simulink model "smc"  (R2022b)
settings: Solver=VariableStepAuto  StartTime=0.0  StopTime=10
undefined symbols (not defined in the file or in its folder): a, beta, d1, d2, delta, DZ, I, km, miu, wb, wcp, wm
settings Model: Creator=andre  LastModifiedBy=felip
settings SolverCC: ZeroCrossAlgorithm=Adaptive  AlgebraicLoopSolver=TrustRegion
settings DebuggingCC: IgnoredZcDiagnostic=none  UnconnectedInputMsg=warning  UnconnectedOutputMsg=warning  UnconnectedLineMsg=warning  SFMachineParentedDataDiag=warning
settings ModelReferenceCC: EnableRefExpFcnMdlSchedulingChecks=on
settings RTWCC: DLArmComputeVersion=19.05

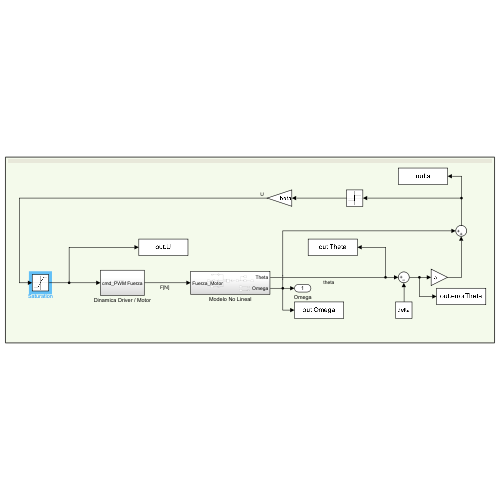
[thumbnail: Simulink's stored preview of the top-level diagram]
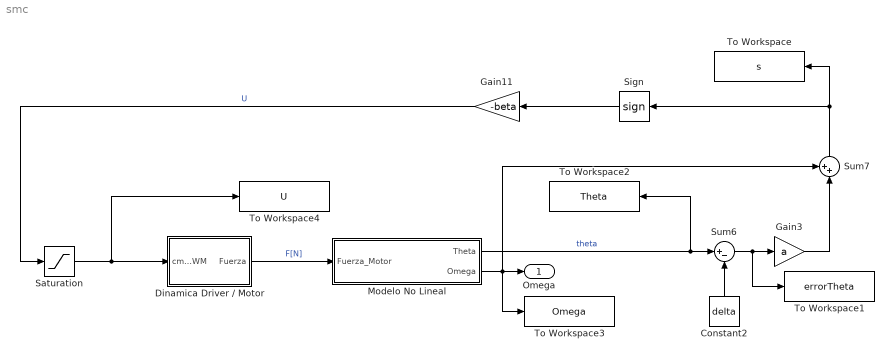
== system smc ==
  Constant2 : Constant  Value=delta
  Dinamica Driver / Motor : Subsystem
  Gain11 : Gain  Gain=-beta
  Gain3 : Gain  Gain=a
  Modelo No Lineal : Subsystem
  Saturation : Saturate  UpperLimit=95  LowerLimit=5  ZeroCross=off
  Sign : Signum  ZeroCross=off
  Sum6 : Sum  Inputs=|+-
  Sum7 : Sum  Inputs=++|
  To Workspace : ToWorkspace  VariableName=s  SaveFormat=Timeseries  SampleTime=-1
  To Workspace1 : ToWorkspace  VariableName=errorTheta  SaveFormat=Timeseries  SampleTime=-1
  To Workspace2 : ToWorkspace  VariableName=Theta  SaveFormat=Timeseries  SampleTime=-1
  To Workspace3 : ToWorkspace  VariableName=Omega  SaveFormat=Timeseries  SampleTime=-1
  To Workspace4 : ToWorkspace  VariableName=U  SaveFormat=Timeseries  SampleTime=-1
  Omega : Outport
  wires:
  Gain3/1 -> Sum7/2
  Modelo No Lineal/1(Theta) -> To Workspace2/1, Sum6/1  "theta"
  Sum7/1 -> To Workspace/1, Sign/1
  Gain11/1 -> Saturation/1  "U"
  Constant2/1 -> Sum6/2
  Dinamica Driver / Motor/1(Fuerza) -> Modelo No Lineal/1(Fuerza_Motor)  "F[N]"
  Modelo No Lineal/2(Omega) -> To Workspace3/1, Omega/1, Sum7/1
  Saturation/1 -> To Workspace4/1, Dinamica Driver / Motor/1(cmd_PWM)
  Sign/1 -> Gain11/1
  Sum6/1 -> To Workspace1/1, Gain3/1

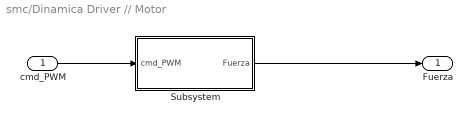
== system smc/Dinamica Driver // Motor ==
  cmd_PWM : Inport
  Subsystem : Subsystem
  Fuerza : Outport
  wires:
  Subsystem/1(Fuerza) -> Fuerza/1
  cmd_PWM/1 -> Subsystem/1(cmd_PWM)

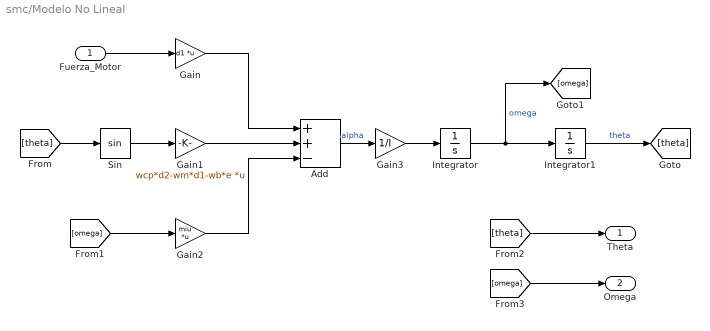
== system smc/Modelo No Lineal ==
  Fuerza_Motor : Inport
  Add : Sum  Inputs=++-
  Gain : Gain  Gain=d1  Multiplication=Matrix(K*u)
  Gain1 : Gain  Gain=wcp*d2-wm*d1-wb*e  Multiplication=Matrix(K*u)
  Gain2 : Gain  Gain=miu  Multiplication=Matrix(K*u)
  Gain3 : Gain  Gain=1/I
  Integrator : Integrator  ZeroCross=off
  Integrator1 : Integrator  ZeroCross=off
  Sin : Trigonometry  ApproximationMethod=CORDIC  NumberOfIterations=13
  Theta : Outport
  Omega : Outport  Port=2
  wires:
  [omega] -> Omega/1
  Gain1/1 -> Add/2
  Integrator/1 -> [omega], Integrator1/1  "omega"
  Fuerza_Motor/1 -> Gain/1
  Integrator1/1 -> [theta]  "theta"
  Gain2/1 -> Add/3
  Gain/1 -> Add/1
  Add/1 -> Gain3/1  "alpha"
  [theta] -> Sin/1
  [omega] -> Gain2/1
  [theta] -> Theta/1
  Sin/1 -> Gain1/1
  Gain3/1 -> Integrator/1

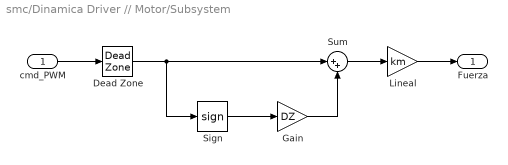
== system smc/Dinamica Driver // Motor/Subsystem ==
  cmd_PWM : Inport
  Dead Zone : DeadZone  LowerValue=-DZ  UpperValue=DZ  ZeroCross=off
  Gain : Gain  Gain=DZ
  Lineal : Gain  Gain=km
  Sign : Signum  ZeroCross=off
  Sum : Sum  Inputs=|++
  Fuerza : Outport
  wires:
  cmd_PWM/1 -> Dead Zone/1
  Dead Zone/1 -> Sum/1, Sign/1
  Sum/1 -> Lineal/1
  Sign/1 -> Gain/1
  Gain/1 -> Sum/2
  Lineal/1 -> Fuerza/1
